simulink model "Wind_AC_PM_Generator"  (R2022a)
settings: Solver=FixedStepAuto  StartTime=0.0  StopTime=Setpoint.PLL.Tsim  FixedStep=Tsc  RelTol=1e-3  EnableMultiTasking=on
PreLoadFcn:
  | %ee_pm_generator_battery_charging_data
InitFcn:
  | ee_pm_generator_battery_charging_data;
StopFcn:
  | ee_addSimlogTimeStamp(bdroot)
undefined symbols (not defined in the file or in its folder): Electric, Ld, Lq, p, Plate, psim, R_h2, Setpoint, Tsc
libraries: fl_lib x34, nesl_utility x21, ee_lib x10, eeTransforms x2, eePmsmCurrentController x1, eeGeneralControl x1, slpidlib x1, eePwmGeneratorTwoLevel x1, spsRMSLib x1
(part 5 of 5)

== system Wind_AC_PM_Generator/Control Unit/Field Oriented Control/Outer loop control/Subsystem ==
  N : Inport
  1-D Lookup Table : Lookup_n-D  NumberOfTableDimensions=1  BreakpointsForDimension1=[500 1000]  Table=[480 640]  InternalRulePriority=Speed  RndMeth=Simplest
  Rate Limiter : RateLimiter  RisingSlewLimit=500/1  FallingSlewLimit=-500/1  SampleTimeMode=inherited
  vdc_set : Outport
  wires:
  1-D Lookup Table/1 -> vdc_set/1  "vdc_set"
  Rate Limiter/1 -> 1-D Lookup Table/1
  N/1 -> Rate Limiter/1

== matlab function Wind_AC_PM_Generator/Electrolyzer/Sensor/MATLAB Function ==
  data: u input; Z output
function Z = fcn(u)

Z = min(u(2)/u(1),1e3);
